simulink model "pendulum"  (R2016b)
settings: Solver=ode45  StartTime=0.0  StopTime=43  FixedStep=0.1  RelTol=1e-12  EnableMultiTasking=on
settings Model: Creator=amal029_old  LastModifiedBy=amal029_old
settings SolverCC: ZeroCrossAlgorithm=Adaptive  AutoInsertRateTranBlk=on
settings DataIOCC: LimitDataPoints=on
settings OptimizationCC: LifeSpan=inf
settings DebuggingCC: AllowSymbolicDim=off  SFUnexpectedBacktrackingDiag=warning  SFNoUnconditionalDefaultTransitionDiag=warning  SFExecutionAtInitializationDiag=none
settings GRTTargetCC: TargetLangStandard=C89/C90 (ANSI)
settings ConfigComp: CovMetricSettings=dw  CovHtmlReporting=on  CovSaveCumulativeToWorkspaceVar=on  CovSaveSingleToWorkspaceVar=on  CovShowResultsExplorer=off  CovExternalEMLEnable=off

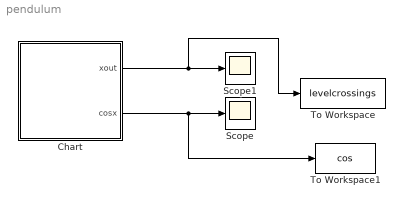
== system pendulum ==
  Chart : Stateflow chart  TreatAsAtomicUnit=on
  Scope : Scope
  Scope1 : Scope
  To Workspace : ToWorkspace  VariableName=levelcrossings  SaveFormat=Timeseries  SampleTime=-1
  To Workspace1 : ToWorkspace  VariableName=cos  SaveFormat=Timeseries  SampleTime=-1
  wires:
  Chart/1(xout) -> To Workspace/1, Scope1/1
  Chart/2(cosx) -> To Workspace1/1, Scope/1

== stateflow chart pendulum/Chart ==
  settings: updateMethod=CONTINUOUS
  state State2
    du:
    x_dot=-0.4;
    xout=x;
    cosx=cos(x);
  state State1
    du:
    x_dot=0.1;
    xout = x;
    cosx=cos(x);
    % Max step-size = 10^-2
  State1 -> State2 : [cos(x) <= -0.99]
  State2 -> State1 : [cos(x) >= 0.99]
  (default) -> State1 : {x=9*pi/2; cosx=cos(x); xout=x;}
  data: x local; xout output; cosx output
  data x settings: updateMethod=SF_CONTINUOUS_TIME_DATA
